simulink model "Ayush-Main_Data_Flow"  (R2023a)
settings: Solver=FixedStepAuto  StartTime=0.0  StopTime=10.0  FixedStep=1e-3  RelTol=1e-3  EnableMultiTasking=on
undefined symbols (not defined in the file): D0, D1, D10, D11, D12, D13, D14, D15, D2, D3, D4, D5, D6, D7, D8, D9, PTA0, PTA1, PTA2, PTB23, PTB9, PTC16, PTC17, PTC2, PTC3, PTC4, PTD0, PTD1, PTD2, PTD3, PTE24, PTE25
libraries: frdmk64flib x16
settings Model: ExtModeTrigDuration=5  Creator=sadeg  LastModifiedBy=ayush
settings OptimizationCC: EnhancedBackFolding=on  PassReuseOutputArgsAs=Individual arguments  ZeroExternalMemoryAtStartup=off  ZeroInternalMemoryAtStartup=off  MaxStackSize=64  OptimizeBlockOrder=speed  DifferentSizesBufferReuse=on  OptimizationCustomize=off  EfficientTunableParamExpr=on
settings DebuggingCC: ParameterTunabilityLossMsg=error
settings HardwareCC: ProdBitPerPointer=32  ProdBitPerSizeT=32  ProdBitPerPtrDiffT=32  ProdLargestAtomicInteger=Long  ProdLargestAtomicFloat=Double  ProdWordSize=32  ProdHWDeviceType=ARM Compatible->ARM Cortex  UseEmbeddedCoderFeatures=off
settings SFSimCC: MATLABDynamicMemAlloc=off
settings RTWCC: Description=Embedded Coder  SystemTargetFile=ert.tlc  HardwareBoard=NXP FRDM-K64F  TLCOptions="-aInlineSetEventsForThisBaseRateFcn=TLC_FALSE -aSuppressMultiTaskScheduler=TLC_FALSE  -aRateBasedStepFcn=0"  TemplateMakefile=ert_default_tmf  Toolchain=GNU Tools for ARM Embedded Processors
settings CodeAppCC: ForceParamTrailComments=on  IgnoreCustomStorageClasses=off  OperatorAnnotations=on  SimulinkDataObjDesc=on  SFDataObjDesc=on  InsertBlockDesc=on
settings ERTTargetCC: SupportNonInlinedSFcns=on  ExtModeTransport=4  ExtModeMexFile=sendToCommService

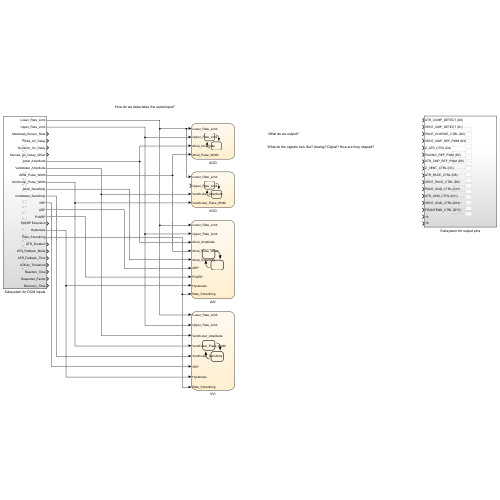
[thumbnail: Simulink's stored preview of the top-level diagram]
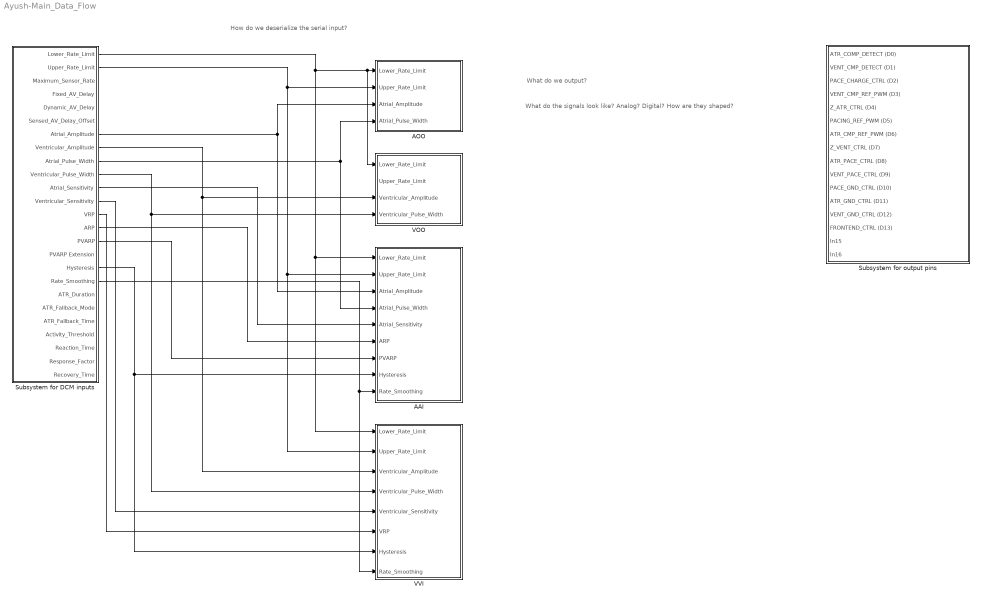
== system Ayush-Main_Data_Flow ==
  note: What do the signals look like? Analog? Digital? How are they shaped?
  note: What do we output?
  note: How do we deserialize the serial input?
  AAI : Stateflow chart  TreatAsAtomicUnit=on
  AOO : Stateflow chart  TreatAsAtomicUnit=on
  Subsystem for DCM inputs : Subsystem
  Subsystem for output pins : Subsystem
  VOO : Stateflow chart  TreatAsAtomicUnit=on
  VVI : Stateflow chart  TreatAsAtomicUnit=on
  wires:
  Subsystem for DCM inputs/1(Lower_Rate_Limit) -> VVI/1(Lower_Rate_Limit), AAI/1(Lower_Rate_Limit), VOO/1(Lower_Rate_Limit), AOO/1(Lower_Rate_Limit)
  Subsystem for DCM inputs/2(Upper_Rate_Limit) -> VVI/2(Upper_Rate_Limit), AAI/2(Upper_Rate_Limit), AOO/2(Upper_Rate_Limit)
  Subsystem for DCM inputs/7(Atrial_Amplitude) -> AAI/3(Atrial_Amplitude), AOO/3(Atrial_Amplitude)
  Subsystem for DCM inputs/9(Atrial_Pulse_Width) -> AAI/4(Atrial_Pulse_Width), AOO/4(Atrial_Pulse_Width)
  Subsystem for DCM inputs/8(Ventricular_Amplitude) -> VVI/3(Ventricular_Amplitude), VOO/3(Ventricular_Amplitude)
  Subsystem for DCM inputs/10(Ventricular_Pulse_Width) -> VVI/4(Ventricular_Pulse_Width), VOO/4(Ventricular_Pulse_Width)
  Subsystem for DCM inputs/11(Atrial_Sensitivity) -> AAI/5(Atrial_Sensitivity)
  Subsystem for DCM inputs/14(ARP) -> AAI/6(ARP)
  Subsystem for DCM inputs/15(PVARP) -> AAI/7(PVARP)
  Subsystem for DCM inputs/17(Hysteresis) -> VVI/7(Hysteresis), AAI/8(Hysteresis)
  Subsystem for DCM inputs/18(Rate_Smoothing) -> VVI/8(Rate_Smoothing), AAI/9(Rate_Smoothing)
  Subsystem for DCM inputs/12(Ventricular_Sensitivity) -> VVI/5(Ventricular_Sensitivity)
  Subsystem for DCM inputs/13(VRP) -> VVI/6(VRP)

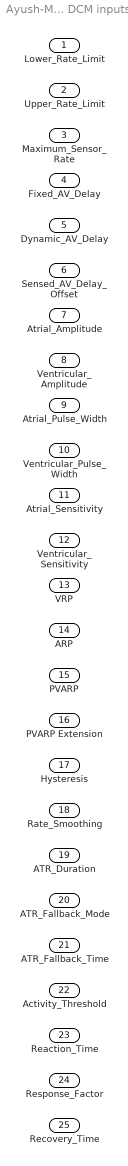
== system Ayush-Main_Data_Flow/Subsystem for DCM inputs ==
  Lower_Rate_Limit : Outport
  Upper_Rate_Limit : Outport  Port=2
  Maximum_Sensor_Rate : Outport  Port=3
  Fixed_AV_Delay : Outport  Port=4
  Dynamic_AV_Delay : Outport  Port=5
  Sensed_AV_Delay_Offset : Outport  Port=6
  Atrial_Amplitude : Outport  Port=7
  Ventricular_Amplitude : Outport  Port=8
  Atrial_Pulse_Width : Outport  Port=9
  Ventricular_Pulse_Width : Outport  Port=10
  Atrial_Sensitivity : Outport  Port=11
  Ventricular_Sensitivity : Outport  Port=12
  VRP : Outport  Port=13
  ARP : Outport  Port=14
  PVARP : Outport  Port=15
  PVARP Extension : Outport  Port=16
  Hysteresis : Outport  Port=17
  Rate_Smoothing : Outport  Port=18
  ATR_Duration : Outport  Port=19
  ATR_Fallback_Mode : Outport  Port=20
  ATR_Fallback_Time : Outport  Port=21
  Activity_Threshold : Outport  Port=22
  Reaction_Time : Outport  Port=23
  Response_Factor : Outport  Port=24
  Recovery_Time : Outport  Port=25

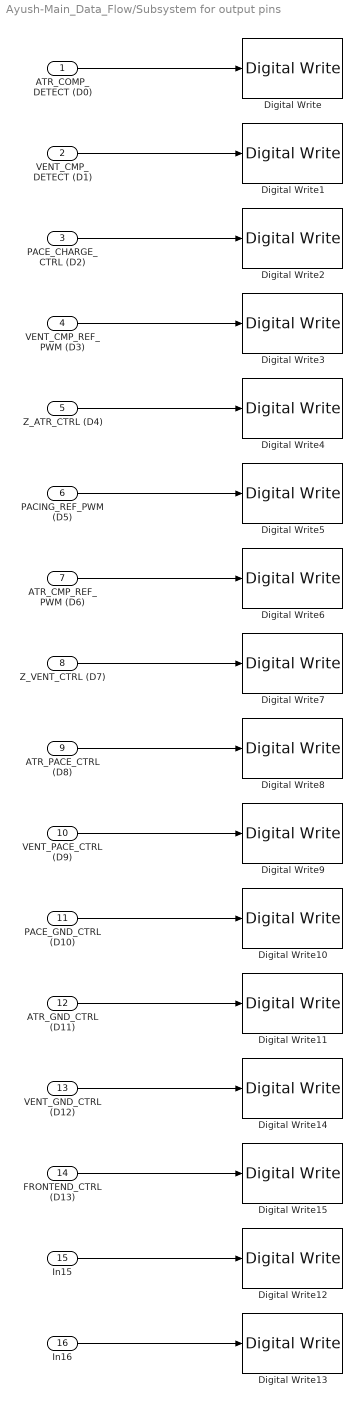
== system Ayush-Main_Data_Flow/Subsystem for output pins ==
  ATR_COMP_DETECT (D0) : Inport
  VENT_CMP_DETECT (D1) : Inport  Port=2
  PACE_CHARGE_CTRL (D2) : Inport  Port=3
  VENT_CMP_REF_PWM (D3) : Inport  Port=4
  Z_ATR_CTRL (D4) : Inport  Port=5
  PACING_REF_PWM (D5) : Inport  Port=6
  ATR_CMP_REF_PWM (D6) : Inport  Port=7
  Z_VENT_CTRL (D7) : Inport  Port=8
  ATR_PACE_CTRL (D8) : Inport  Port=9
  VENT_PACE_CTRL (D9) : Inport  Port=10
  PACE_GND_CTRL (D10) : Inport  Port=11
  ATR_GND_CTRL (D11) : Inport  Port=12
  VENT_GND_CTRL (D12) : Inport  Port=13
  FRONTEND_CTRL (D13) : Inport  Port=14
  In15 : Inport  Port=15
  In16 : Inport  Port=16
  Digital Write : frdmk64flib/Digital Write  Whichpin=PTC16 (D0)
  Digital Write1 : frdmk64flib/Digital Write  Whichpin=PTC17 (D1)
  Digital Write10 : frdmk64flib/Digital Write  Whichpin=PTD0 (D10)
  Digital Write11 : frdmk64flib/Digital Write  Whichpin=PTD2 (D11)
  Digital Write12 : frdmk64flib/Digital Write  Whichpin=PTE25 (D14)
  Digital Write13 : frdmk64flib/Digital Write  Whichpin=PTE24 (D15)
  Digital Write14 : frdmk64flib/Digital Write  Whichpin=PTD3 (D12)
  Digital Write15 : frdmk64flib/Digital Write  Whichpin=PTD1 (D13)
  Digital Write2 : frdmk64flib/Digital Write  Whichpin=PTB9 (D2)
  Digital Write3 : frdmk64flib/Digital Write  Whichpin=PTA1 (D3)
  Digital Write4 : frdmk64flib/Digital Write  Whichpin=PTB23 (D4)
  Digital Write5 : frdmk64flib/Digital Write  Whichpin=PTA2 (D5)
  Digital Write6 : frdmk64flib/Digital Write  Whichpin=PTC2 (D6)
  Digital Write7 : frdmk64flib/Digital Write  Whichpin=PTC3 (D7)
  Digital Write8 : frdmk64flib/Digital Write  Whichpin=PTA0 (D8)
  Digital Write9 : frdmk64flib/Digital Write  Whichpin=PTC4 (D9)
  wires:
  ATR_COMP_DETECT (D0)/1 -> Digital Write/1
  VENT_CMP_DETECT (D1)/1 -> Digital Write1/1
  PACE_CHARGE_CTRL (D2)/1 -> Digital Write2/1
  Z_ATR_CTRL (D4)/1 -> Digital Write4/1
  VENT_CMP_REF_PWM (D3)/1 -> Digital Write3/1
  PACING_REF_PWM (D5)/1 -> Digital Write5/1
  Z_VENT_CTRL (D7)/1 -> Digital Write7/1
  ATR_CMP_REF_PWM (D6)/1 -> Digital Write6/1
  PACE_GND_CTRL (D10)/1 -> Digital Write10/1
  ATR_GND_CTRL (D11)/1 -> Digital Write11/1
  ATR_PACE_CTRL (D8)/1 -> Digital Write8/1
  VENT_PACE_CTRL (D9)/1 -> Digital Write9/1
  In15/1 -> Digital Write12/1
  VENT_GND_CTRL (D12)/1 -> Digital Write14/1
  FRONTEND_CTRL (D13)/1 -> Digital Write15/1
  In16/1 -> Digital Write13/1

== stateflow chart Ayush-Main_Data_Flow/VOO ==
  note: VOO mode paces the ventricle at a constant rate regardless of the natural heartbeat
  state PULSE_VENT
    entry:
    PACE_CHARGE_CTRL = 0;
    PACE_GND_CTRL = 1;
    ATR_PACE_CTRL = 0;
    ATR_GND_CTRL = 0;
    Z_ATR_CTRL = 0;
    Z_VENT_CTRL = 0;
    VENT_GND_CTRL = 0;
    VENT_PACE_CTRL = 1;
  state CHARGE
    entry:
    ATR_PACE_CTRL = 0;
    VENT_PACE_CTRL = 0;
    PACING_REF_PWM = Ventricular_Amplitude;
    PACE_CHARGE_CTRL = 1;
  state DISCHARGE
    entry:
    PACE_GND_CTRL = 1;
    VENT_PACE_CTRL = 0;
    Z_ATR_CTRL = 0;
    Z_VENT_CTRL = 0;
    ATR_PACE_CTRL = 0;
    ATR_GND_CTRL = 0;
    VENT_GND_CTRL = 1;
  note: after(Ventricular_Pulse_Width, msec)
  (default) -> CHARGE
  CHARGE -> PULSE_VENT : after(60/(Lower_Rate_Limit+Upper_Rate_Limit/2),sec)
  DISCHARGE -> CHARGE
  PULSE_VENT -> DISCHARGE
  data: Lower_Rate_Limit input; Upper_Rate_Limit input; Ventricular_Amplitude input; Ventricular_Pulse_Width input

== stateflow chart Ayush-Main_Data_Flow/AAI ==
  state CHARGE
    entry:
    ATR_PACE_CTRL = 0;
    PACE_CHARGE_CTRL = 1;
  (default) -> CHARGE
  data: Lower_Rate_Limit input; Upper_Rate_Limit input; Atrial_Amplitude input; Atrial_Pulse_Width input; Atrial_Sensitivity input; ARP input; PVARP input; Hysteresis input; Rate_Smoothing input

== stateflow chart Ayush-Main_Data_Flow/AOO ==
  state PULSE_ATR
    entry:
    PACE_CHARGE_CTRL = 0;
    PACE_GND_CTRL = 1;
    VENT_GND_CTRL = 0;
    VENT_PACE_CTRL = 0;
    Z_ATR_CTRL = 0;
    Z_VENT_CTRL = 0;
    ATR_GND_CTRL = 0;
    ATR_PACE_CTRL = 1;
  state CHARGE
    entry:
    ATR_PACE_CTRL = 0;
    VENT_PACE_CTRL = 0;
    PACING_REF_PWM = Atrial_Amplitude;
    PACE_CHARGE_CTRL = 1;
  state DISCHARGE
    entry:
    PACE_GND_CTRL = 1;
    VENT_PACE_CTRL = 0;
    Z_ATR_CTRL = 0;
    Z_VENT_CTRL = 0;
    ATR_PACE_CTRL = 0;
    ATR_GND_CTRL = 0;
    VENT_GND_CTRL = 1;
  (default) -> CHARGE
  CHARGE -> PULSE_ATR : after(60/(Lower_Rate_Limit+Upper_Rate_Limit/2),sec)
  DISCHARGE -> CHARGE
  PULSE_ATR -> DISCHARGE : after(Atrial_Pulse_Width, msec)
  data: Lower_Rate_Limit input; Upper_Rate_Limit input; Atrial_Amplitude input; Atrial_Pulse_Width input

== stateflow chart Ayush-Main_Data_Flow/VVI ==
  data: Lower_Rate_Limit input; Upper_Rate_Limit input; Ventricular_Amplitude input; Ventricular_Pulse_Width input; Ventricular_Sensitivity input; VRP input; Hysteresis input; Rate_Smoothing input
